simulink model "T5_button_controllable"  (R2022b)
settings: Solver=FixedStepAuto  StartTime=0.0  StopTime=96  FixedStep=0.01  RelTol=1e-3
undefined symbols (not defined in the file): cableArea, High, Low, Scaling_factor, Ts, Vnom
libraries: fl_lib x145, nesl_utility x56, simulink x54, ee_lib x4
(part 1 of 3)
settings Model: Creator=mingreico  LastModifiedBy=mingreico

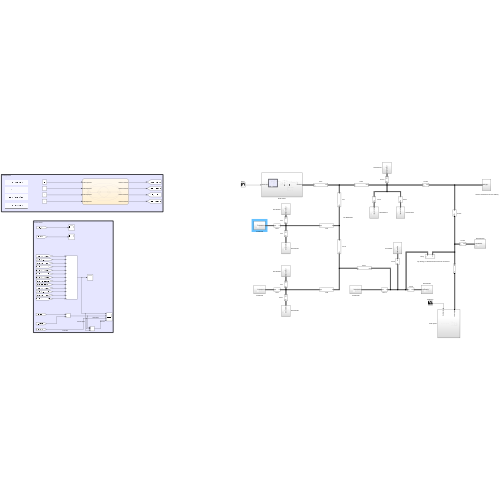
[thumbnail: Simulink's stored preview of the top-level diagram]
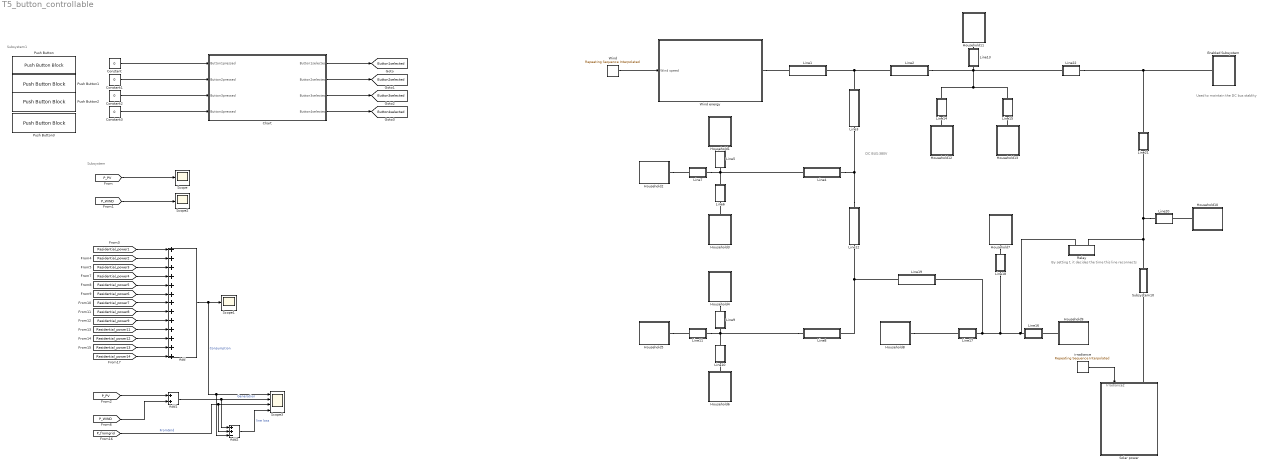
== system T5_button_controllable ==
  note: Subsystem
  note: Subsystem1
  note: By setting t, it decides the time this line reconnects
  note: Used to maintain the DC bus stablity
  note: DC BUS:380V
  Add : Sum  Inputs=+++++++++++++
  Add1 : Sum
  Add2 : Sum  Inputs=++-
  Chart : Stateflow chart  TreatAsAtomicUnit=on
  Constant{,1..3} (4 alike) : Constant  Value=0  OutDataTypeStr=boolean
  Enabled Subsystem : Subsystem
  Household1 : Subsystem
  Household10 : Subsystem
  Household11 : Subsystem
  Household12 : Subsystem
  Household13 : Subsystem
  Household2 : Subsystem
  Household3 : Subsystem
  Household4 : Subsystem
  Household5 : Subsystem
  Household6 : Subsystem
  Household7 : Subsystem
  Household8 : Subsystem
  Household9 : Subsystem
  Line1 : Subsystem  mask{rho=1.68e-8, l=2.0, A=cableArea}
      mask prompts: rho "Specific resistivity in Ohm*m"; l "Length in m"; A "Cross sectional area in m^2"
  Line10 : Subsystem  mask{rho=1.68e-8, l=2.0, A=cableArea}
      mask prompts: rho "Specific resistivity in Ohm*m"; l "Length in m"; A "Cross sectional area in m^2"
  Line11 : Subsystem  mask{rho=1.68e-8, l=2.0, A=cableArea}
      mask prompts: rho "Specific resistivity in Ohm*m"; l "Length in m"; A "Cross sectional area in m^2"
  Line12 : Subsystem  mask{rho=1.68e-8, l=2.0, A=cableArea}
      mask prompts: rho "Specific resistivity in Ohm*m"; l "Length in m"; A "Cross sectional area in m^2"
  Line13 : Subsystem  mask{rho=1.68e-8, l=2.0, A=cableArea}
      mask prompts: rho "Specific resistivity in Ohm*m"; l "Length in m"; A "Cross sectional area in m^2"
  Line14 : Subsystem  mask{rho=1.68e-8, l=2.0, A=cableArea}
      mask prompts: rho "Specific resistivity in Ohm*m"; l "Length in m"; A "Cross sectional area in m^2"
  Line15 : Subsystem  mask{rho=1.68e-8, l=2.0, A=cableArea}
      mask prompts: rho "Specific resistivity in Ohm*m"; l "Length in m"; A "Cross sectional area in m^2"
  Line16 : Subsystem  mask{rho=1.68e-8, l=2.0, A=cableArea}
      mask prompts: rho "Specific resistivity in Ohm*m"; l "Length in m"; A "Cross sectional area in m^2"
  Line17 : Subsystem  mask{rho=1.68e-8, l=2.0, A=cableArea}
      mask prompts: rho "Specific resistivity in Ohm*m"; l "Length in m"; A "Cross sectional area in m^2"
  Line18 : Subsystem  mask{rho=1.68e-8, l=2.0, A=cableArea}
      mask prompts: rho "Specific resistivity in Ohm*m"; l "Length in m"; A "Cross sectional area in m^2"
  Line19 : Subsystem  mask{rho=1.68e-8, l=2.0, A=cableArea}
      mask prompts: rho "Specific resistivity in Ohm*m"; l "Length in m"; A "Cross sectional area in m^2"
  Line2 : Subsystem  mask{rho=1.68e-8, l=2.0, A=cableArea}
      mask prompts: rho "Specific resistivity in Ohm*m"; l "Length in m"; A "Cross sectional area in m^2"
  Line20 : Subsystem  mask{rho=1.68e-8, l=2.0, A=cableArea}
      mask prompts: rho "Specific resistivity in Ohm*m"; l "Length in m"; A "Cross sectional area in m^2"
  Line21 : Subsystem  mask{rho=1.68e-8, l=2.0, A=cableArea}
      mask prompts: rho "Specific resistivity in Ohm*m"; l "Length in m"; A "Cross sectional area in m^2"
  Line22 : Subsystem  mask{rho=1.68e-8, l=2.0, A=cableArea}
      mask prompts: rho "Specific resistivity in Ohm*m"; l "Length in m"; A "Cross sectional area in m^2"
  Line3 : Subsystem  mask{rho=1.68e-8, l=2.0, A=cableArea}
      mask prompts: rho "Specific resistivity in Ohm*m"; l "Length in m"; A "Cross sectional area in m^2"
  Line4 : Subsystem  mask{rho=1.68e-8, l=2.0, A=cableArea}
      mask prompts: rho "Specific resistivity in Ohm*m"; l "Length in m"; A "Cross sectional area in m^2"
  Line5 : Subsystem  mask{rho=1.68e-8, l=2.0, A=cableArea}
      mask prompts: rho "Specific resistivity in Ohm*m"; l "Length in m"; A "Cross sectional area in m^2"
  Line6 : Subsystem  mask{rho=1.68e-8, l=2.0, A=cableArea}
      mask prompts: rho "Specific resistivity in Ohm*m"; l "Length in m"; A "Cross sectional area in m^2"
  Line7 : Subsystem  mask{rho=1.68e-8, l=2.0, A=cableArea}
      mask prompts: rho "Specific resistivity in Ohm*m"; l "Length in m"; A "Cross sectional area in m^2"
  Line8 : Subsystem  mask{rho=1.68e-8, l=2.0, A=cableArea}
      mask prompts: rho "Specific resistivity in Ohm*m"; l "Length in m"; A "Cross sectional area in m^2"
  Line9 : Subsystem  mask{rho=1.68e-8, l=2.0, A=cableArea}
      mask prompts: rho "Specific resistivity in Ohm*m"; l "Length in m"; A "Cross sectional area in m^2"
  Push Button : PushButtonBlock  ButtonText=Button_SpringAllday  OffValue=0.000000
  Push Button1 : PushButtonBlock  ButtonText=Button_SummerAllday  OffValue=0.000000
  Push Button2 : PushButtonBlock  ButtonText=Button_AutumnAllday  OffValue=0.000000
  Push Button3 : PushButtonBlock  ButtonText=Button_WinterAllday  OffValue=0.000000
  Relay : Subsystem  mask{t=140}
      mask prompts: t "Specific jumping time"
  Scope : Scope
  Scope1 : Scope
  Scope2 : Scope
  Scope3 : Scope  NumInputPorts=4
  Solar power : Subsystem
  Subsystem10 : Subsystem  mask{rho=1.68e-8, l=2.0, A=cableArea}
      mask prompts: rho "Specific resistivity in Ohm*m"; l "Length in m"; A "Cross sectional area in m^2"
  "Wind  " : simulink/Sources/Repeating Sequence Interpolated  OutValues=[6 5 5 8 10 11 17 20 22 29 31 36 34 37 37 37 32 30 29 22 15 11 9 13]*0.7  TimeValues=[0 1 2 3 4 5 6 7 8 9 10 11 12 13 14 15 16 17 18 19 20 21 22 23]  LookUpMeth=Interpolation-Use End Values  tsamp=0.01  OutMin=[]  OutMax=[]  OutDataTypeStr=double  OutputDataTypeScalingMode=double  OutDataType=fixdt(0,8)  OutScaling=2^-10
  Wind energy : Subsystem
  "irradiance " : simulink/Sources/Repeating Sequence Interpolated  OutValues=[0 0 0 0 0 0 43 163 310 464 601 707 776 810 807 769 696 594 469 331 189 52 0 0]  TimeValues=[0 1 2 3 4 5 6 7 8 9 10 11 12 13 14 15 16 17 18 19 20 21 22 23]  LookUpMeth=Interpolation-Use End Values  tsamp=0.01  OutMin=[]  OutMax=[]  OutDataTypeStr=double  OutputDataTypeScalingMode=double  OutDataType=fixdt(0,8)  OutScaling=2^-10
  tag scope: Button1selected=global, Button2selected=global, Button3selected=global, Button4selected=global
  wires:
  Constant3/1 -> Chart/4(Button4pressed)
  Constant2/1 -> Chart/3(Button3pressed)
  Constant1/1 -> Chart/2(Button2pressed)
  Constant/1 -> Chart/1(Button1pressed)
  Chart/4(" Button4selected") -> [Button4selected]
  Chart/3(" Button3selected") -> [Button3selected]
  Chart/2(" Button2selected") -> [Button2selected]
  Chart/1(" Button1selected") -> [Button1selected]
  Add1/1 -> Add2/1, Scope3/2  "Generation"
  [P_WIND] -> Add1/2
  [P_PV] -> Add1/1
  Add/1 -> Scope1/1, Add2/3, Scope3/1  "Consumption"
  [Residential_power13] -> Add/12
  [Residential_power12] -> Add/11
  [Residential_power11] -> Add/10
  [Residential_power9] -> Add/9
  [Residential_power8] -> Add/8
  [Residential_power7] -> Add/7
  [Residential_power6] -> Add/6
  [Residential_power5] -> Add/5
  [Residential_power4] -> Add/4
  [Residential_power3] -> Add/3
  [Residential_power2] -> Add/2
  [Residential_power1] -> Add/1
  [P_WIND] -> Scope2/1
  [P_PV] -> Scope/1
  [P_fromgrid] -> Add2/2, Scope3/3  "FromGrid"
  [Residential_power14] -> Add/13
  Add2/1 -> Scope3/4  "line loss"
  "irradiance "/1 -> Solar power/1(Irradiance2)
  "Wind  "/1 -> Wind energy/1(Wind speed)
  connections:
  Line8/RConn1 -- Line9/LConn1 -- Line10/RConn1 -- Line11/LConn1
  Line2/RConn1 -- Line14/LConn1 -- Line15/LConn1 -- Line22/LConn1 -- Line13/LConn1
  Line20/LConn1 -- Relay/LConn2 -- Subsystem10/RConn1 -- Line21/RConn1
  Line1/RConn1 -- Line2/LConn1 -- Line3/LConn1
  Line8/LConn1 -- Line12/RConn1 -- Line19/LConn1
  Line16/LConn1 -- Line18/LConn1 -- Line17/LConn1 -- Line19/RConn1 -- Relay/LConn1
  Line21/LConn1 -- Enabled Subsystem/RConn1 -- Line22/RConn1
  Line12/LConn1 -- Line3/RConn1 -- Line4/LConn1
  Line7/LConn1 -- Line5/LConn1 -- Line4/RConn1 -- Line6/RConn1
  Household12/RConn1 -- Line14/RConn1
  Household1/RConn1 -- Line5/RConn1
  Household13/RConn1 -- Line15/RConn1
  Household7/RConn1 -- Line18/RConn1
  Household6/RConn1 -- Line10/LConn1
  Household9/RConn1 -- Line16/RConn1
  Household8/RConn1 -- Line17/RConn1
  Household11/RConn1 -- Line13/RConn1
  Household5/RConn1 -- Line11/RConn1
  Household2/RConn1 -- Line7/RConn1
  Household4/RConn1 -- Line9/RConn1
  Household3/RConn1 -- Line6/LConn1
  Household10/RConn1 -- Line20/RConn1
  Wind energy/RConn1 -- Line1/LConn1
  Solar power/LConn1 -- Subsystem10/LConn1

== system T5_button_controllable/Enabled Subsystem ==
  Average-Value DC-DC Converter : ee_lib/Semiconductors & Converters/Converters/Average-Value DC-DC Converter  control_option=ee.enum.converters.controlinput.voltage  converter_type=ee.enum.converters.dcdctype.buck  efficiency_option=ee.enum.converters.efficiency.constant  efficiency_fixed=100  i_vec=[0, 2, 5] A  efficiency_vec=[90, 95, 98]
      settings: InternalSimscapePortConfiguration="{\"Bottom\":[],\"Left\":[{\"id\":\"Vref\",\"label\":\"Vref\",\"type\":\"input\"},{\"id\":\"p1\",\"label\":\"1+\",\"type\":\"foundation.electrical.electrical\"},{\"id\":\"n1\",\"label\":\"1-\",\"type\":\"foundation.electrical.electrical\"}],\"Right\":[{\"id\":\"p2\",\"label\":\"2+\",\"type\":\"foundation.electrical.electrical\"},{\"id\":\"n2\",\"label\":\"2-\",\"type\":\"foundation.electrical.electrical\"}],\"Top\":[]}"
  Constant : Constant  Value=Vnom
  Current Sensor : fl_lib/Electrical/Electrical Sensors/Current Sensor
  PS-Simulink Converter : nesl_utility/PS-Simulink Converter  PhysicalDomain=network_engine_domain  SubClassName=ps_output  LeftPortType=input  RightPortType=output  PseudoPeriodic=off  Frequencies=[]  VectorFormat=inherit  Unit=inherit  AffineConversion=off
  PS-Simulink Converter1 : nesl_utility/PS-Simulink Converter  PhysicalDomain=network_engine_domain  SubClassName=ps_output  LeftPortType=input  RightPortType=output  PseudoPeriodic=off  Frequencies=[]  VectorFormat=inherit  Unit=inherit  AffineConversion=off
  Product : Product
  Scope : Scope
  Simscape Bus1 : SimscapeBus  HierarchyStrings=High;Low
  Simulink-PS Converter : nesl_utility/Simulink-PS Converter  PhysicalDomain=network_engine_domain  SubClassName=ps_input  LeftPortType=input  RightPortType=output  PseudoPeriodic=off  Frequencies=[]  NoiseDistribution=none  NoiseParameters=[]  Unit=1  AffineConversion=off  FilteringAndDerivatives=provide  SimscapeFilterOrder=1  InputFilterTimeConstant=0.001  UdotUserProvided=0
  Voltage Sensor : fl_lib/Electrical/Electrical Sensors/Voltage Sensor
  Voltage Source : ee_lib/Sources/Voltage Source  dc_voltage=1000 V  ac_voltage=0 V  ac_shift=0 rad  ac_frequency=60 Hz  noise_mode=ee.enum.sources.noise.Disabled  PSD=0 V^2/Hz  sample_time=1e-3 s  repeatability=ee.enum.sources.repeatability.NotRepeatable  user_seed=0  auto_seed=3499211588  i_specify=off  i_priority=None  i=0 A  i_nominal_specify=off  i_nominal_unit=A  i_nominal_value=1  v_specify=off  v_priority=None  v=0 V  v_nominal_specify=off  v_nominal_unit=V  v_nominal_value=1
  Maingrid : PMIOPort  Side=Right
  tag scope: P_fromgrid=global
  wires:
  Constant/1 -> Simulink-PS Converter/1
  PS-Simulink Converter/1 -> Scope/1, Product/1
  PS-Simulink Converter1/1 -> Product/2
  Product/1 -> [P_fromgrid]
  connections:
  Maingrid/RConn1 -- Simscape Bus1/RConn1
  Voltage Source/LConn1 -- Average-Value DC-DC Converter/LConn2
  Voltage Source/RConn1 -- Average-Value DC-DC Converter/LConn3
  Simulink-PS Converter/RConn1 -- Average-Value DC-DC Converter/LConn1
  Average-Value DC-DC Converter/RConn2 -- Voltage Sensor/RConn2 -- Simscape Bus1/LConn2
  Current Sensor/RConn2 -- Voltage Sensor/LConn1 -- Simscape Bus1/LConn1
  Current Sensor/LConn1 -- Average-Value DC-DC Converter/RConn1
  PS-Simulink Converter1/LConn1 -- Voltage Sensor/RConn1
  PS-Simulink Converter/LConn1 -- Current Sensor/RConn1

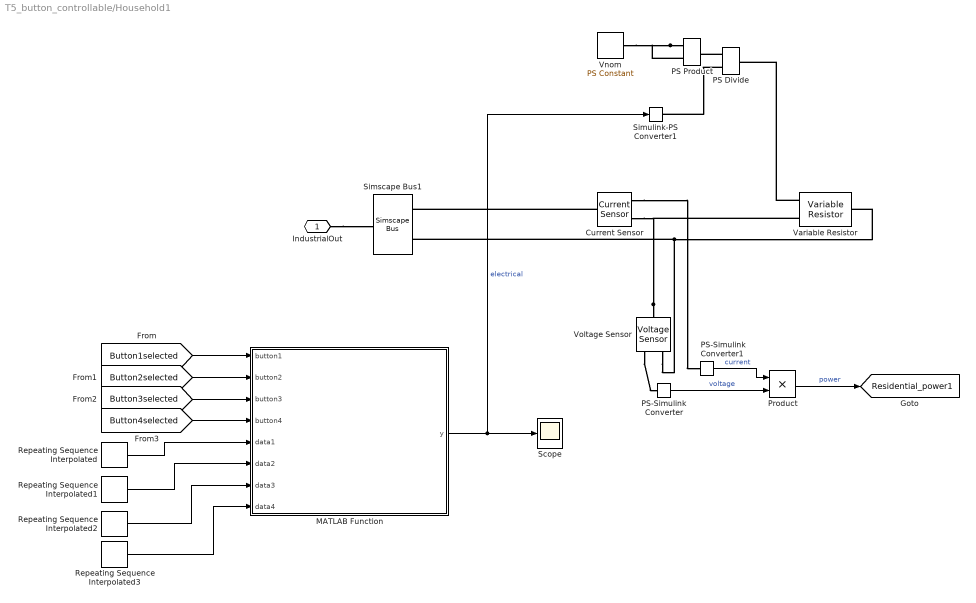
== system T5_button_controllable/Household1 ==
  Current Sensor : fl_lib/Electrical/Electrical Sensors/Current Sensor
  MATLAB Function : MATLAB Function  TreatAsAtomicUnit=on
  PS Divide : fl_lib/Physical Signals/Functions/PS Divide
  PS Product : fl_lib/Physical Signals/Functions/PS Product
  PS-Simulink Converter : nesl_utility/PS-Simulink Converter  PhysicalDomain=network_engine_domain  SubClassName=ps_output  LeftPortType=input  RightPortType=output  PseudoPeriodic=off  Frequencies=[]  VectorFormat=inherit  Unit=inherit  AffineConversion=off
  PS-Simulink Converter1 : nesl_utility/PS-Simulink Converter  PhysicalDomain=network_engine_domain  SubClassName=ps_output  LeftPortType=input  RightPortType=output  PseudoPeriodic=off  Frequencies=[]  VectorFormat=inherit  Unit=inherit  AffineConversion=off
  Product : Product
  Repeating Sequence Interpolated : simulink/Sources/Repeating Sequence Interpolated  OutValues=Household3_Springallday  TimeValues=Allday_timevector  LookUpMeth=Interpolation-Use End Values  tsamp=0.01  OutMin=[]  OutMax=[]  OutDataTypeStr=double  OutputDataTypeScalingMode=double  OutDataType=fixdt(0,8)  OutScaling=2^-10
  Repeating Sequence Interpolated1 : simulink/Sources/Repeating Sequence Interpolated  OutValues=Household3_Summerallday  TimeValues=Allday_timevector  LookUpMeth=Interpolation-Use End Values  tsamp=0.01  OutMin=[]  OutMax=[]  OutDataTypeStr=double  OutputDataTypeScalingMode=double  OutDataType=fixdt(0,8)  OutScaling=2^-10
  Repeating Sequence Interpolated2 : simulink/Sources/Repeating Sequence Interpolated  OutValues=Household3_Autumnallday  TimeValues=Allday_timevector  LookUpMeth=Interpolation-Use End Values  tsamp=0.01  OutMin=[]  OutMax=[]  OutDataTypeStr=double  OutputDataTypeScalingMode=double  OutDataType=fixdt(0,8)  OutScaling=2^-10
  Repeating Sequence Interpolated3 : simulink/Sources/Repeating Sequence Interpolated  OutValues=Household3_Winterallday  TimeValues=Allday_timevector  LookUpMeth=Interpolation-Use End Values  tsamp=0.01  OutMin=[]  OutMax=[]  OutDataTypeStr=double  OutputDataTypeScalingMode=double  OutDataType=fixdt(0,8)  OutScaling=2^-10
  Scope : Scope
  Simscape Bus1 : SimscapeBus  HierarchyStrings=High;Low
  Simulink-PS Converter1 : nesl_utility/Simulink-PS Converter  PhysicalDomain=network_engine_domain  SubClassName=ps_input  LeftPortType=input  RightPortType=output  PseudoPeriodic=off  Frequencies=[]  NoiseDistribution=none  NoiseParameters=[]  Unit=V*A  AffineConversion=off  FilteringAndDerivatives=provide  SimscapeFilterOrder=1  InputFilterTimeConstant=0.001  UdotUserProvided=0
  Variable Resistor : fl_lib/Electrical/Electrical Elements/Variable Resistor  Rmin=0 Ohm  i_specify=off  i_priority=None  i=0 A  i_nominal_specify=off  i_nominal_unit=A  i_nominal_value=1  v_specify=off  v_priority=None  v=0 V  v_nominal_specify=off  v_nominal_unit=V  v_nominal_value=1
  Vnom : fl_lib/Physical Signals/Sources/PS Constant  constant=Vnom V
  Voltage Sensor : fl_lib/Electrical/Electrical Sensors/Voltage Sensor
  IndustrialOut : PMIOPort  Side=Right
  tag scope: Residential_power1=global
  wires:
  MATLAB Function/1(y) -> Simulink-PS Converter1/1, Scope/1  "electrical"
  PS-Simulink Converter/1 -> Product/2  "voltage"
  PS-Simulink Converter1/1 -> Product/1  "current"
  Product/1 -> [Residential_power1]  "power"
  [Button4selected] -> MATLAB Function/4(button4)
  [Button3selected] -> MATLAB Function/3(button3)
  [Button2selected] -> MATLAB Function/2(button2)
  [Button1selected] -> MATLAB Function/1(button1)
  Repeating Sequence Interpolated/1 -> MATLAB Function/5(data1)
  Repeating Sequence Interpolated1/1 -> MATLAB Function/6(data2)
  Repeating Sequence Interpolated2/1 -> MATLAB Function/7(data3)
  Repeating Sequence Interpolated3/1 -> MATLAB Function/8(data4)
  connections:
  PS Divide/LConn1 -- PS Product/RConn1
  Variable Resistor/LConn1 -- PS Divide/RConn1
  PS Divide/LConn2 -- Simulink-PS Converter1/RConn1
  PS Product/LConn1 -- PS Product/LConn2 -- Vnom/RConn1
  Voltage Sensor/RConn2 -- Variable Resistor/RConn1 -- Simscape Bus1/LConn2
  IndustrialOut/RConn1 -- Simscape Bus1/RConn1
  Voltage Sensor/LConn1 -- Variable Resistor/LConn2 -- Current Sensor/RConn2
  Voltage Sensor/RConn1 -- PS-Simulink Converter/LConn1
  Current Sensor/RConn1 -- PS-Simulink Converter1/LConn1
  Current Sensor/LConn1 -- Simscape Bus1/LConn1

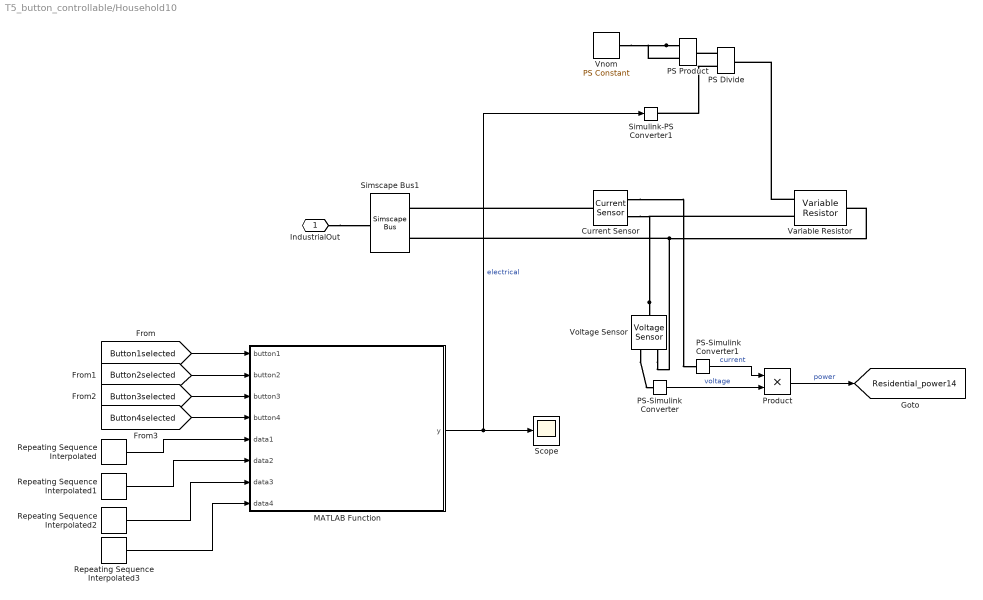
== system T5_button_controllable/Household10 ==
  Current Sensor : fl_lib/Electrical/Electrical Sensors/Current Sensor
  MATLAB Function : MATLAB Function  TreatAsAtomicUnit=on
  PS Divide : fl_lib/Physical Signals/Functions/PS Divide
  PS Product : fl_lib/Physical Signals/Functions/PS Product
  PS-Simulink Converter : nesl_utility/PS-Simulink Converter  PhysicalDomain=network_engine_domain  SubClassName=ps_output  LeftPortType=input  RightPortType=output  PseudoPeriodic=off  Frequencies=[]  VectorFormat=inherit  Unit=inherit  AffineConversion=off
  PS-Simulink Converter1 : nesl_utility/PS-Simulink Converter  PhysicalDomain=network_engine_domain  SubClassName=ps_output  LeftPortType=input  RightPortType=output  PseudoPeriodic=off  Frequencies=[]  VectorFormat=inherit  Unit=inherit  AffineConversion=off
  Product : Product
  Repeating Sequence Interpolated : simulink/Sources/Repeating Sequence Interpolated  OutValues=Household14_Springallday  TimeValues=Allday_timevector  LookUpMeth=Interpolation-Use End Values  tsamp=0.01  OutMin=[]  OutMax=[]  OutDataTypeStr=double  OutputDataTypeScalingMode=double  OutDataType=fixdt(0,8)  OutScaling=2^-10
  Repeating Sequence Interpolated1 : simulink/Sources/Repeating Sequence Interpolated  OutValues=Household14_Summerallday  TimeValues=Allday_timevector  LookUpMeth=Interpolation-Use End Values  tsamp=0.01  OutMin=[]  OutMax=[]  OutDataTypeStr=double  OutputDataTypeScalingMode=double  OutDataType=fixdt(0,8)  OutScaling=2^-10
  Repeating Sequence Interpolated2 : simulink/Sources/Repeating Sequence Interpolated  OutValues=Household14_Autumnallday  TimeValues=Allday_timevector  LookUpMeth=Interpolation-Use End Values  tsamp=0.01  OutMin=[]  OutMax=[]  OutDataTypeStr=double  OutputDataTypeScalingMode=double  OutDataType=fixdt(0,8)  OutScaling=2^-10
  Repeating Sequence Interpolated3 : simulink/Sources/Repeating Sequence Interpolated  OutValues=Household14_Winterallday  TimeValues=Allday_timevector  LookUpMeth=Interpolation-Use End Values  tsamp=0.01  OutMin=[]  OutMax=[]  OutDataTypeStr=double  OutputDataTypeScalingMode=double  OutDataType=fixdt(0,8)  OutScaling=2^-10
  Scope : Scope
  Simscape Bus1 : SimscapeBus  HierarchyStrings=High;Low
  Simulink-PS Converter1 : nesl_utility/Simulink-PS Converter  PhysicalDomain=network_engine_domain  SubClassName=ps_input  LeftPortType=input  RightPortType=output  PseudoPeriodic=off  Frequencies=[]  NoiseDistribution=none  NoiseParameters=[]  Unit=V*A  AffineConversion=off  FilteringAndDerivatives=provide  SimscapeFilterOrder=1  InputFilterTimeConstant=0.001  UdotUserProvided=0
  Variable Resistor : fl_lib/Electrical/Electrical Elements/Variable Resistor  Rmin=0 Ohm  i_specify=off  i_priority=None  i=0 A  i_nominal_specify=off  i_nominal_unit=A  i_nominal_value=1  v_specify=off  v_priority=None  v=0 V  v_nominal_specify=off  v_nominal_unit=V  v_nominal_value=1
  Vnom : fl_lib/Physical Signals/Sources/PS Constant  constant=Vnom V
  Voltage Sensor : fl_lib/Electrical/Electrical Sensors/Voltage Sensor
  IndustrialOut : PMIOPort  Side=Right
  tag scope: Residential_power14=global
  wires:
  MATLAB Function/1(y) -> Scope/1, Simulink-PS Converter1/1  "electrical"
  PS-Simulink Converter/1 -> Product/2  "voltage"
  PS-Simulink Converter1/1 -> Product/1  "current"
  Product/1 -> [Residential_power14]  "power"
  [Button4selected] -> MATLAB Function/4(button4)
  [Button3selected] -> MATLAB Function/3(button3)
  [Button2selected] -> MATLAB Function/2(button2)
  [Button1selected] -> MATLAB Function/1(button1)
  Repeating Sequence Interpolated/1 -> MATLAB Function/5(data1)
  Repeating Sequence Interpolated1/1 -> MATLAB Function/6(data2)
  Repeating Sequence Interpolated2/1 -> MATLAB Function/7(data3)
  Repeating Sequence Interpolated3/1 -> MATLAB Function/8(data4)
  connections:
  PS Divide/LConn1 -- PS Product/RConn1
  Variable Resistor/LConn1 -- PS Divide/RConn1
  PS Divide/LConn2 -- Simulink-PS Converter1/RConn1
  PS Product/LConn1 -- PS Product/LConn2 -- Vnom/RConn1
  Voltage Sensor/RConn2 -- Simscape Bus1/LConn2 -- Variable Resistor/RConn1
  IndustrialOut/RConn1 -- Simscape Bus1/RConn1
  Voltage Sensor/LConn1 -- Variable Resistor/LConn2 -- Current Sensor/RConn2
  Voltage Sensor/RConn1 -- PS-Simulink Converter/LConn1
  Current Sensor/RConn1 -- PS-Simulink Converter1/LConn1
  Current Sensor/LConn1 -- Simscape Bus1/LConn1

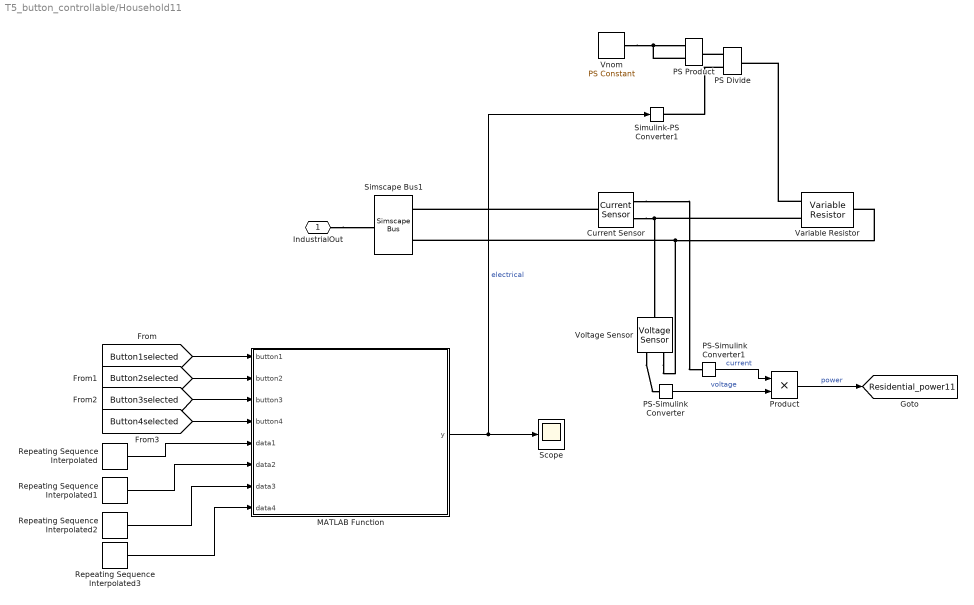
== system T5_button_controllable/Household11 ==
  Current Sensor : fl_lib/Electrical/Electrical Sensors/Current Sensor
  MATLAB Function : MATLAB Function  TreatAsAtomicUnit=on
  PS Divide : fl_lib/Physical Signals/Functions/PS Divide
  PS Product : fl_lib/Physical Signals/Functions/PS Product
  PS-Simulink Converter : nesl_utility/PS-Simulink Converter  PhysicalDomain=network_engine_domain  SubClassName=ps_output  LeftPortType=input  RightPortType=output  PseudoPeriodic=off  Frequencies=[]  VectorFormat=inherit  Unit=inherit  AffineConversion=off
  PS-Simulink Converter1 : nesl_utility/PS-Simulink Converter  PhysicalDomain=network_engine_domain  SubClassName=ps_output  LeftPortType=input  RightPortType=output  PseudoPeriodic=off  Frequencies=[]  VectorFormat=inherit  Unit=inherit  AffineConversion=off
  Product : Product
  Repeating Sequence Interpolated : simulink/Sources/Repeating Sequence Interpolated  OutValues=Household7_Springallday  TimeValues=Allday_timevector  LookUpMeth=Interpolation-Use End Values  tsamp=0.01  OutMin=[]  OutMax=[]  OutDataTypeStr=double  OutputDataTypeScalingMode=double  OutDataType=fixdt(0,8)  OutScaling=2^-10
  Repeating Sequence Interpolated1 : simulink/Sources/Repeating Sequence Interpolated  OutValues=Household7_Summerallday  TimeValues=Allday_timevector  LookUpMeth=Interpolation-Use End Values  tsamp=0.01  OutMin=[]  OutMax=[]  OutDataTypeStr=double  OutputDataTypeScalingMode=double  OutDataType=fixdt(0,8)  OutScaling=2^-10
  Repeating Sequence Interpolated2 : simulink/Sources/Repeating Sequence Interpolated  OutValues=Household7_Autumnallday  TimeValues=Allday_timevector  LookUpMeth=Interpolation-Use End Values  tsamp=0.01  OutMin=[]  OutMax=[]  OutDataTypeStr=double  OutputDataTypeScalingMode=double  OutDataType=fixdt(0,8)  OutScaling=2^-10
  Repeating Sequence Interpolated3 : simulink/Sources/Repeating Sequence Interpolated  OutValues=Household7_Winterallday  TimeValues=Allday_timevector  LookUpMeth=Interpolation-Use End Values  tsamp=0.01  OutMin=[]  OutMax=[]  OutDataTypeStr=double  OutputDataTypeScalingMode=double  OutDataType=fixdt(0,8)  OutScaling=2^-10
  Scope : Scope
  Simscape Bus1 : SimscapeBus  HierarchyStrings=High;Low
  Simulink-PS Converter1 : nesl_utility/Simulink-PS Converter  PhysicalDomain=network_engine_domain  SubClassName=ps_input  LeftPortType=input  RightPortType=output  PseudoPeriodic=off  Frequencies=[]  NoiseDistribution=none  NoiseParameters=[]  Unit=V*A  AffineConversion=off  FilteringAndDerivatives=provide  SimscapeFilterOrder=1  InputFilterTimeConstant=0.001  UdotUserProvided=0
  Variable Resistor : fl_lib/Electrical/Electrical Elements/Variable Resistor  Rmin=0 Ohm  i_specify=off  i_priority=None  i=0 A  i_nominal_specify=off  i_nominal_unit=A  i_nominal_value=1  v_specify=off  v_priority=None  v=0 V  v_nominal_specify=off  v_nominal_unit=V  v_nominal_value=1
  Vnom : fl_lib/Physical Signals/Sources/PS Constant  constant=Vnom V
  Voltage Sensor : fl_lib/Electrical/Electrical Sensors/Voltage Sensor
  IndustrialOut : PMIOPort  Side=Right
  tag scope: Residential_power11=global
  wires:
  Repeating Sequence Interpolated3/1 -> MATLAB Function/8(data4)
  Repeating Sequence Interpolated2/1 -> MATLAB Function/7(data3)
  Repeating Sequence Interpolated1/1 -> MATLAB Function/6(data2)
  Repeating Sequence Interpolated/1 -> MATLAB Function/5(data1)
  [Button1selected] -> MATLAB Function/1(button1)
  [Button2selected] -> MATLAB Function/2(button2)
  [Button3selected] -> MATLAB Function/3(button3)
  [Button4selected] -> MATLAB Function/4(button4)
  Product/1 -> [Residential_power11]  "power"
  PS-Simulink Converter1/1 -> Product/1  "current"
  PS-Simulink Converter/1 -> Product/2  "voltage"
  MATLAB Function/1(y) -> Simulink-PS Converter1/1, Scope/1  "electrical"
  connections:
  Current Sensor/LConn1 -- Simscape Bus1/LConn1
  Current Sensor/RConn1 -- PS-Simulink Converter1/LConn1
  Voltage Sensor/RConn1 -- PS-Simulink Converter/LConn1
  Current Sensor/RConn2 -- Variable Resistor/LConn2 -- Voltage Sensor/LConn1
  IndustrialOut/RConn1 -- Simscape Bus1/RConn1
  Variable Resistor/RConn1 -- Simscape Bus1/LConn2 -- Voltage Sensor/RConn2
  Vnom/RConn1 -- PS Product/LConn2 -- PS Product/LConn1
  PS Divide/LConn2 -- Simulink-PS Converter1/RConn1
  Variable Resistor/LConn1 -- PS Divide/RConn1
  PS Divide/LConn1 -- PS Product/RConn1

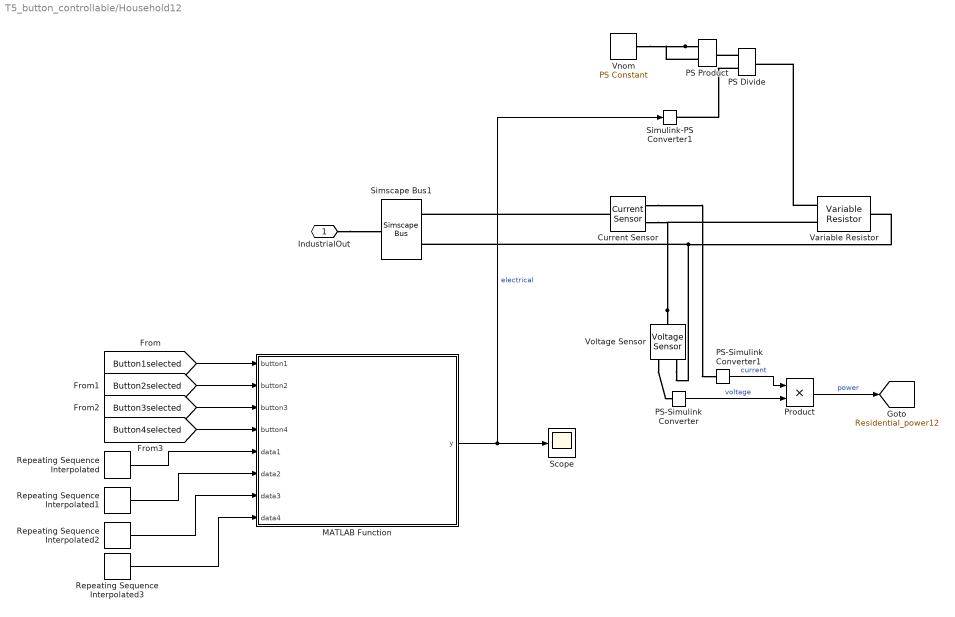
== system T5_button_controllable/Household12 ==
  Current Sensor : fl_lib/Electrical/Electrical Sensors/Current Sensor
  MATLAB Function : MATLAB Function  TreatAsAtomicUnit=on
  PS Divide : fl_lib/Physical Signals/Functions/PS Divide
  PS Product : fl_lib/Physical Signals/Functions/PS Product
  PS-Simulink Converter : nesl_utility/PS-Simulink Converter  PhysicalDomain=network_engine_domain  SubClassName=ps_output  LeftPortType=input  RightPortType=output  PseudoPeriodic=off  Frequencies=[]  VectorFormat=inherit  Unit=inherit  AffineConversion=off
  PS-Simulink Converter1 : nesl_utility/PS-Simulink Converter  PhysicalDomain=network_engine_domain  SubClassName=ps_output  LeftPortType=input  RightPortType=output  PseudoPeriodic=off  Frequencies=[]  VectorFormat=inherit  Unit=inherit  AffineConversion=off
  Product : Product
  Repeating Sequence Interpolated : simulink/Sources/Repeating Sequence Interpolated  OutValues=Household11_Springallday  TimeValues=Allday_timevector  LookUpMeth=Interpolation-Use End Values  tsamp=0.01  OutMin=[]  OutMax=[]  OutDataTypeStr=double  OutputDataTypeScalingMode=double  OutDataType=fixdt(0,8)  OutScaling=2^-10
  Repeating Sequence Interpolated1 : simulink/Sources/Repeating Sequence Interpolated  OutValues=Household11_Summerallday  TimeValues=Allday_timevector  LookUpMeth=Interpolation-Use End Values  tsamp=0.01  OutMin=[]  OutMax=[]  OutDataTypeStr=double  OutputDataTypeScalingMode=double  OutDataType=fixdt(0,8)  OutScaling=2^-10
  Repeating Sequence Interpolated2 : simulink/Sources/Repeating Sequence Interpolated  OutValues=Household11_Autumnallday  TimeValues=Allday_timevector  LookUpMeth=Interpolation-Use End Values  tsamp=0.01  OutMin=[]  OutMax=[]  OutDataTypeStr=double  OutputDataTypeScalingMode=double  OutDataType=fixdt(0,8)  OutScaling=2^-10
  Repeating Sequence Interpolated3 : simulink/Sources/Repeating Sequence Interpolated  OutValues=Household11_Winterallday  TimeValues=Allday_timevector  LookUpMeth=Interpolation-Use End Values  tsamp=0.01  OutMin=[]  OutMax=[]  OutDataTypeStr=double  OutputDataTypeScalingMode=double  OutDataType=fixdt(0,8)  OutScaling=2^-10
  Scope : Scope
  Simscape Bus1 : SimscapeBus  HierarchyStrings=High;Low
  Simulink-PS Converter1 : nesl_utility/Simulink-PS Converter  PhysicalDomain=network_engine_domain  SubClassName=ps_input  LeftPortType=input  RightPortType=output  PseudoPeriodic=off  Frequencies=[]  NoiseDistribution=none  NoiseParameters=[]  Unit=V*A  AffineConversion=off  FilteringAndDerivatives=provide  SimscapeFilterOrder=1  InputFilterTimeConstant=0.001  UdotUserProvided=0
  Variable Resistor : fl_lib/Electrical/Electrical Elements/Variable Resistor  Rmin=0 Ohm  i_specify=off  i_priority=None  i=0 A  i_nominal_specify=off  i_nominal_unit=A  i_nominal_value=1  v_specify=off  v_priority=None  v=0 V  v_nominal_specify=off  v_nominal_unit=V  v_nominal_value=1
  Vnom : fl_lib/Physical Signals/Sources/PS Constant  constant=Vnom V
  Voltage Sensor : fl_lib/Electrical/Electrical Sensors/Voltage Sensor
  IndustrialOut : PMIOPort  Side=Right
  tag scope: Residential_power12=global
  wires:
  MATLAB Function/1(y) -> Simulink-PS Converter1/1, Scope/1  "electrical"
  PS-Simulink Converter/1 -> Product/2  "voltage"
  PS-Simulink Converter1/1 -> Product/1  "current"
  Product/1 -> [Residential_power12]  "power"
  [Button4selected] -> MATLAB Function/4(button4)
  [Button3selected] -> MATLAB Function/3(button3)
  [Button2selected] -> MATLAB Function/2(button2)
  [Button1selected] -> MATLAB Function/1(button1)
  Repeating Sequence Interpolated/1 -> MATLAB Function/5(data1)
  Repeating Sequence Interpolated1/1 -> MATLAB Function/6(data2)
  Repeating Sequence Interpolated2/1 -> MATLAB Function/7(data3)
  Repeating Sequence Interpolated3/1 -> MATLAB Function/8(data4)
  connections:
  PS Divide/LConn1 -- PS Product/RConn1
  Variable Resistor/LConn1 -- PS Divide/RConn1
  PS Divide/LConn2 -- Simulink-PS Converter1/RConn1
  PS Product/LConn1 -- PS Product/LConn2 -- Vnom/RConn1
  Voltage Sensor/RConn2 -- Simscape Bus1/LConn2 -- Variable Resistor/RConn1
  IndustrialOut/RConn1 -- Simscape Bus1/RConn1
  Voltage Sensor/LConn1 -- Variable Resistor/LConn2 -- Current Sensor/RConn2
  Voltage Sensor/RConn1 -- PS-Simulink Converter/LConn1
  Current Sensor/RConn1 -- PS-Simulink Converter1/LConn1
  Current Sensor/LConn1 -- Simscape Bus1/LConn1

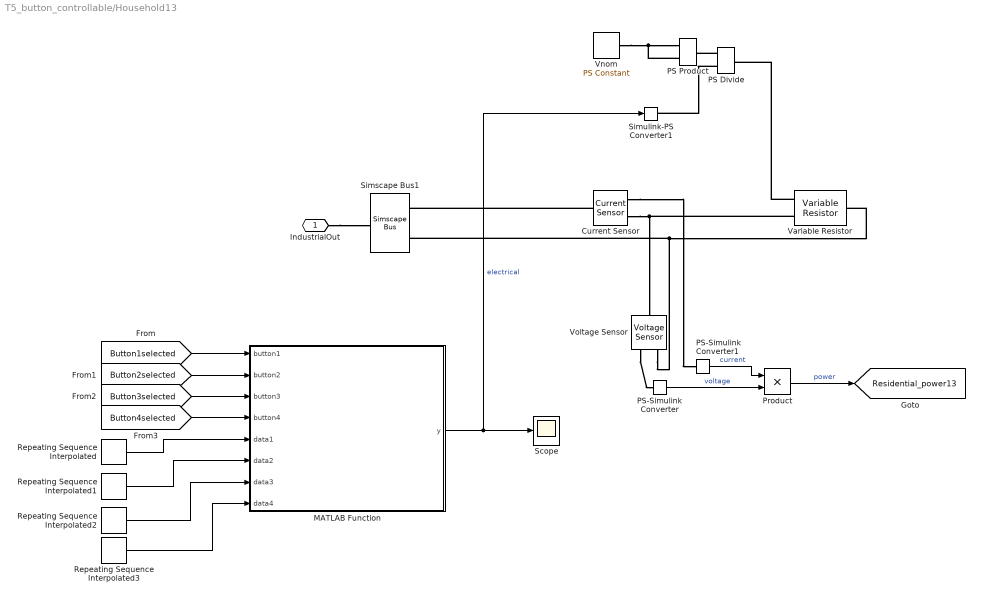
== system T5_button_controllable/Household13 ==
  Current Sensor : fl_lib/Electrical/Electrical Sensors/Current Sensor
  MATLAB Function : MATLAB Function  TreatAsAtomicUnit=on
  PS Divide : fl_lib/Physical Signals/Functions/PS Divide
  PS Product : fl_lib/Physical Signals/Functions/PS Product
  PS-Simulink Converter : nesl_utility/PS-Simulink Converter  PhysicalDomain=network_engine_domain  SubClassName=ps_output  LeftPortType=input  RightPortType=output  PseudoPeriodic=off  Frequencies=[]  VectorFormat=inherit  Unit=inherit  AffineConversion=off
  PS-Simulink Converter1 : nesl_utility/PS-Simulink Converter  PhysicalDomain=network_engine_domain  SubClassName=ps_output  LeftPortType=input  RightPortType=output  PseudoPeriodic=off  Frequencies=[]  VectorFormat=inherit  Unit=inherit  AffineConversion=off
  Product : Product
  Repeating Sequence Interpolated : simulink/Sources/Repeating Sequence Interpolated  OutValues=Household12_Springallday  TimeValues=Allday_timevector  LookUpMeth=Interpolation-Use End Values  tsamp=0.01  OutMin=[]  OutMax=[]  OutDataTypeStr=double  OutputDataTypeScalingMode=double  OutDataType=fixdt(0,8)  OutScaling=2^-10
  Repeating Sequence Interpolated1 : simulink/Sources/Repeating Sequence Interpolated  OutValues=Household12_Summerallday  TimeValues=Allday_timevector  LookUpMeth=Interpolation-Use End Values  tsamp=0.01  OutMin=[]  OutMax=[]  OutDataTypeStr=double  OutputDataTypeScalingMode=double  OutDataType=fixdt(0,8)  OutScaling=2^-10
  Repeating Sequence Interpolated2 : simulink/Sources/Repeating Sequence Interpolated  OutValues=Household12_Autumnallday  TimeValues=Allday_timevector  LookUpMeth=Interpolation-Use End Values  tsamp=0.01  OutMin=[]  OutMax=[]  OutDataTypeStr=double  OutputDataTypeScalingMode=double  OutDataType=fixdt(0,8)  OutScaling=2^-10
  Repeating Sequence Interpolated3 : simulink/Sources/Repeating Sequence Interpolated  OutValues=Household12_Winterallday  TimeValues=Allday_timevector  LookUpMeth=Interpolation-Use End Values  tsamp=0.01  OutMin=[]  OutMax=[]  OutDataTypeStr=double  OutputDataTypeScalingMode=double  OutDataType=fixdt(0,8)  OutScaling=2^-10
  Scope : Scope
  Simscape Bus1 : SimscapeBus  HierarchyStrings=High;Low
  Simulink-PS Converter1 : nesl_utility/Simulink-PS Converter  PhysicalDomain=network_engine_domain  SubClassName=ps_input  LeftPortType=input  RightPortType=output  PseudoPeriodic=off  Frequencies=[]  NoiseDistribution=none  NoiseParameters=[]  Unit=V*A  AffineConversion=off  FilteringAndDerivatives=provide  SimscapeFilterOrder=1  InputFilterTimeConstant=0.001  UdotUserProvided=0
  Variable Resistor : fl_lib/Electrical/Electrical Elements/Variable Resistor  Rmin=0 Ohm  i_specify=off  i_priority=None  i=0 A  i_nominal_specify=off  i_nominal_unit=A  i_nominal_value=1  v_specify=off  v_priority=None  v=0 V  v_nominal_specify=off  v_nominal_unit=V  v_nominal_value=1
  Vnom : fl_lib/Physical Signals/Sources/PS Constant  constant=Vnom V
  Voltage Sensor : fl_lib/Electrical/Electrical Sensors/Voltage Sensor
  IndustrialOut : PMIOPort  Side=Right
  tag scope: Residential_power13=global
  wires:
  Repeating Sequence Interpolated3/1 -> MATLAB Function/8(data4)
  Repeating Sequence Interpolated2/1 -> MATLAB Function/7(data3)
  Repeating Sequence Interpolated1/1 -> MATLAB Function/6(data2)
  Repeating Sequence Interpolated/1 -> MATLAB Function/5(data1)
  [Button1selected] -> MATLAB Function/1(button1)
  [Button2selected] -> MATLAB Function/2(button2)
  [Button3selected] -> MATLAB Function/3(button3)
  [Button4selected] -> MATLAB Function/4(button4)
  Product/1 -> [Residential_power13]  "power"
  PS-Simulink Converter1/1 -> Product/1  "current"
  PS-Simulink Converter/1 -> Product/2  "voltage"
  MATLAB Function/1(y) -> Simulink-PS Converter1/1, Scope/1  "electrical"
  connections:
  Current Sensor/LConn1 -- Simscape Bus1/LConn1
  Current Sensor/RConn1 -- PS-Simulink Converter1/LConn1
  Voltage Sensor/RConn1 -- PS-Simulink Converter/LConn1
  Current Sensor/RConn2 -- Variable Resistor/LConn2 -- Voltage Sensor/LConn1
  IndustrialOut/RConn1 -- Simscape Bus1/RConn1
  Variable Resistor/RConn1 -- Simscape Bus1/LConn2 -- Voltage Sensor/RConn2
  Vnom/RConn1 -- PS Product/LConn2 -- PS Product/LConn1
  PS Divide/LConn2 -- Simulink-PS Converter1/RConn1
  Variable Resistor/LConn1 -- PS Divide/RConn1
  PS Divide/LConn1 -- PS Product/RConn1

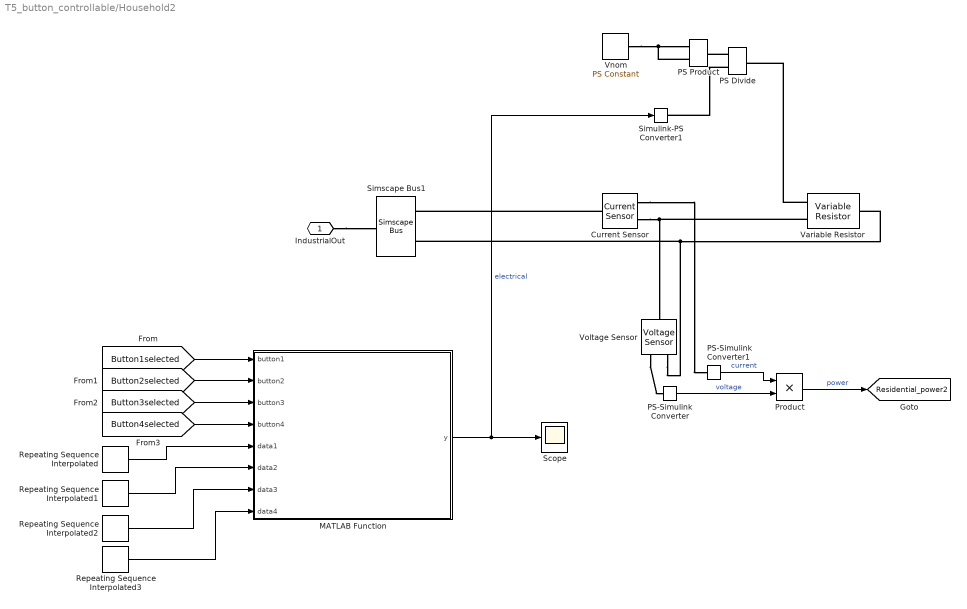
== system T5_button_controllable/Household2 ==
  Current Sensor : fl_lib/Electrical/Electrical Sensors/Current Sensor
  MATLAB Function : MATLAB Function  TreatAsAtomicUnit=on
  PS Divide : fl_lib/Physical Signals/Functions/PS Divide
  PS Product : fl_lib/Physical Signals/Functions/PS Product
  PS-Simulink Converter : nesl_utility/PS-Simulink Converter  PhysicalDomain=network_engine_domain  SubClassName=ps_output  LeftPortType=input  RightPortType=output  PseudoPeriodic=off  Frequencies=[]  VectorFormat=inherit  Unit=inherit  AffineConversion=off
  PS-Simulink Converter1 : nesl_utility/PS-Simulink Converter  PhysicalDomain=network_engine_domain  SubClassName=ps_output  LeftPortType=input  RightPortType=output  PseudoPeriodic=off  Frequencies=[]  VectorFormat=inherit  Unit=inherit  AffineConversion=off
  Product : Product
  Repeating Sequence Interpolated : simulink/Sources/Repeating Sequence Interpolated  OutValues=Household15_Springallday  TimeValues=Allday_timevector  LookUpMeth=Interpolation-Use End Values  tsamp=0.01  OutMin=[]  OutMax=[]  OutDataTypeStr=double  OutputDataTypeScalingMode=double  OutDataType=fixdt(0,8)  OutScaling=2^-10
  Repeating Sequence Interpolated1 : simulink/Sources/Repeating Sequence Interpolated  OutValues=Household15_Summerallday  TimeValues=Allday_timevector  LookUpMeth=Interpolation-Use End Values  tsamp=0.01  OutMin=[]  OutMax=[]  OutDataTypeStr=double  OutputDataTypeScalingMode=double  OutDataType=fixdt(0,8)  OutScaling=2^-10
  Repeating Sequence Interpolated2 : simulink/Sources/Repeating Sequence Interpolated  OutValues=Household15_Autumnallday  TimeValues=Allday_timevector  LookUpMeth=Interpolation-Use End Values  tsamp=0.01  OutMin=[]  OutMax=[]  OutDataTypeStr=double  OutputDataTypeScalingMode=double  OutDataType=fixdt(0,8)  OutScaling=2^-10
  Repeating Sequence Interpolated3 : simulink/Sources/Repeating Sequence Interpolated  OutValues=Household15_Winterallday  TimeValues=Allday_timevector  LookUpMeth=Interpolation-Use End Values  tsamp=0.01  OutMin=[]  OutMax=[]  OutDataTypeStr=double  OutputDataTypeScalingMode=double  OutDataType=fixdt(0,8)  OutScaling=2^-10
  Scope : Scope
  Simscape Bus1 : SimscapeBus  HierarchyStrings=High;Low
  Simulink-PS Converter1 : nesl_utility/Simulink-PS Converter  PhysicalDomain=network_engine_domain  SubClassName=ps_input  LeftPortType=input  RightPortType=output  PseudoPeriodic=off  Frequencies=[]  NoiseDistribution=none  NoiseParameters=[]  Unit=V*A  AffineConversion=off  FilteringAndDerivatives=provide  SimscapeFilterOrder=1  InputFilterTimeConstant=0.001  UdotUserProvided=0
  Variable Resistor : fl_lib/Electrical/Electrical Elements/Variable Resistor  Rmin=0 Ohm  i_specify=off  i_priority=None  i=0 A  i_nominal_specify=off  i_nominal_unit=A  i_nominal_value=1  v_specify=off  v_priority=None  v=0 V  v_nominal_specify=off  v_nominal_unit=V  v_nominal_value=1
  Vnom : fl_lib/Physical Signals/Sources/PS Constant  constant=Vnom V
  Voltage Sensor : fl_lib/Electrical/Electrical Sensors/Voltage Sensor
  IndustrialOut : PMIOPort  Side=Right
  tag scope: Residential_power2=global
  wires:
  Repeating Sequence Interpolated3/1 -> MATLAB Function/8(data4)
  Repeating Sequence Interpolated2/1 -> MATLAB Function/7(data3)
  Repeating Sequence Interpolated1/1 -> MATLAB Function/6(data2)
  Repeating Sequence Interpolated/1 -> MATLAB Function/5(data1)
  [Button1selected] -> MATLAB Function/1(button1)
  [Button2selected] -> MATLAB Function/2(button2)
  [Button3selected] -> MATLAB Function/3(button3)
  [Button4selected] -> MATLAB Function/4(button4)
  Product/1 -> [Residential_power2]  "power"
  PS-Simulink Converter1/1 -> Product/1  "current"
  PS-Simulink Converter/1 -> Product/2  "voltage"
  MATLAB Function/1(y) -> Simulink-PS Converter1/1, Scope/1  "electrical"
  connections:
  Current Sensor/LConn1 -- Simscape Bus1/LConn1
  Current Sensor/RConn1 -- PS-Simulink Converter1/LConn1
  Voltage Sensor/RConn1 -- PS-Simulink Converter/LConn1
  Current Sensor/RConn2 -- Variable Resistor/LConn2 -- Voltage Sensor/LConn1
  IndustrialOut/RConn1 -- Simscape Bus1/RConn1
  Variable Resistor/RConn1 -- Simscape Bus1/LConn2 -- Voltage Sensor/RConn2
  Vnom/RConn1 -- PS Product/LConn2 -- PS Product/LConn1
  PS Divide/LConn2 -- Simulink-PS Converter1/RConn1
  Variable Resistor/LConn1 -- PS Divide/RConn1
  PS Divide/LConn1 -- PS Product/RConn1

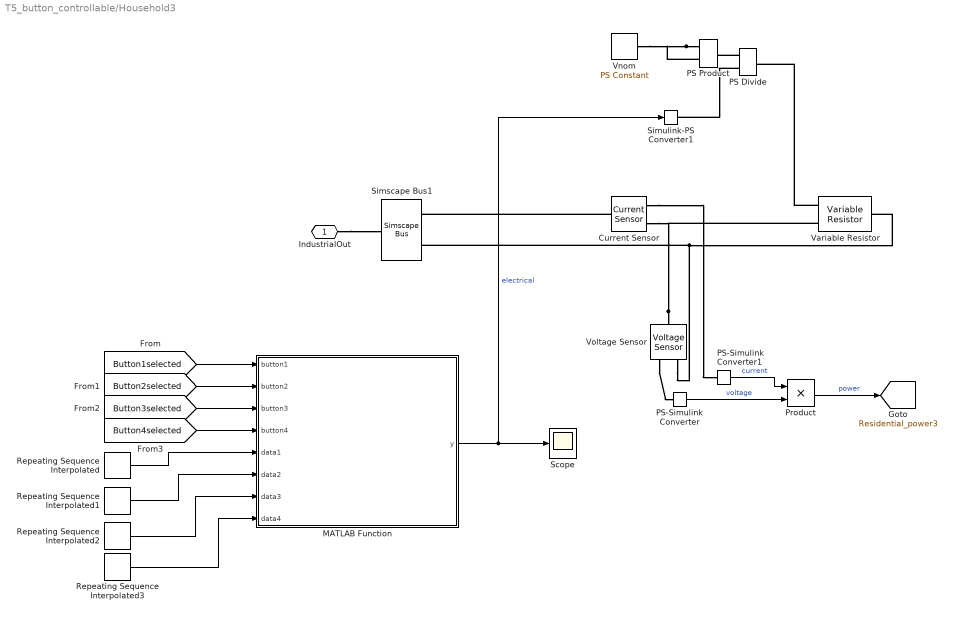
== system T5_button_controllable/Household3 ==
  Current Sensor : fl_lib/Electrical/Electrical Sensors/Current Sensor
  MATLAB Function : MATLAB Function  TreatAsAtomicUnit=on
  PS Divide : fl_lib/Physical Signals/Functions/PS Divide
  PS Product : fl_lib/Physical Signals/Functions/PS Product
  PS-Simulink Converter : nesl_utility/PS-Simulink Converter  PhysicalDomain=network_engine_domain  SubClassName=ps_output  LeftPortType=input  RightPortType=output  PseudoPeriodic=off  Frequencies=[]  VectorFormat=inherit  Unit=inherit  AffineConversion=off
  PS-Simulink Converter1 : nesl_utility/PS-Simulink Converter  PhysicalDomain=network_engine_domain  SubClassName=ps_output  LeftPortType=input  RightPortType=output  PseudoPeriodic=off  Frequencies=[]  VectorFormat=inherit  Unit=inherit  AffineConversion=off
  Product : Product
  Repeating Sequence Interpolated : simulink/Sources/Repeating Sequence Interpolated  OutValues=Household8_Springallday  TimeValues=Allday_timevector  LookUpMeth=Interpolation-Use End Values  tsamp=0.01  OutMin=[]  OutMax=[]  OutDataTypeStr=double  OutputDataTypeScalingMode=double  OutDataType=fixdt(0,8)  OutScaling=2^-10
  Repeating Sequence Interpolated1 : simulink/Sources/Repeating Sequence Interpolated  OutValues=Household8_Summerallday  TimeValues=Allday_timevector  LookUpMeth=Interpolation-Use End Values  tsamp=0.01  OutMin=[]  OutMax=[]  OutDataTypeStr=double  OutputDataTypeScalingMode=double  OutDataType=fixdt(0,8)  OutScaling=2^-10
  Repeating Sequence Interpolated2 : simulink/Sources/Repeating Sequence Interpolated  OutValues=Household8_Autumnallday  TimeValues=Allday_timevector  LookUpMeth=Interpolation-Use End Values  tsamp=0.01  OutMin=[]  OutMax=[]  OutDataTypeStr=double  OutputDataTypeScalingMode=double  OutDataType=fixdt(0,8)  OutScaling=2^-10
  Repeating Sequence Interpolated3 : simulink/Sources/Repeating Sequence Interpolated  OutValues=Household8_Winterallday  TimeValues=Allday_timevector  LookUpMeth=Interpolation-Use End Values  tsamp=0.01  OutMin=[]  OutMax=[]  OutDataTypeStr=double  OutputDataTypeScalingMode=double  OutDataType=fixdt(0,8)  OutScaling=2^-10
  Scope : Scope
  Simscape Bus1 : SimscapeBus  HierarchyStrings=High;Low
  Simulink-PS Converter1 : nesl_utility/Simulink-PS Converter  PhysicalDomain=network_engine_domain  SubClassName=ps_input  LeftPortType=input  RightPortType=output  PseudoPeriodic=off  Frequencies=[]  NoiseDistribution=none  NoiseParameters=[]  Unit=V*A  AffineConversion=off  FilteringAndDerivatives=provide  SimscapeFilterOrder=1  InputFilterTimeConstant=0.001  UdotUserProvided=0
  Variable Resistor : fl_lib/Electrical/Electrical Elements/Variable Resistor  Rmin=0 Ohm  i_specify=off  i_priority=None  i=0 A  i_nominal_specify=off  i_nominal_unit=A  i_nominal_value=1  v_specify=off  v_priority=None  v=0 V  v_nominal_specify=off  v_nominal_unit=V  v_nominal_value=1
  Vnom : fl_lib/Physical Signals/Sources/PS Constant  constant=Vnom V
  Voltage Sensor : fl_lib/Electrical/Electrical Sensors/Voltage Sensor
  IndustrialOut : PMIOPort  Side=Right
  tag scope: Residential_power3=global
  wires:
  MATLAB Function/1(y) -> Simulink-PS Converter1/1, Scope/1  "electrical"
  PS-Simulink Converter/1 -> Product/2  "voltage"
  PS-Simulink Converter1/1 -> Product/1  "current"
  Product/1 -> [Residential_power3]  "power"
  [Button4selected] -> MATLAB Function/4(button4)
  [Button3selected] -> MATLAB Function/3(button3)
  [Button2selected] -> MATLAB Function/2(button2)
  [Button1selected] -> MATLAB Function/1(button1)
  Repeating Sequence Interpolated/1 -> MATLAB Function/5(data1)
  Repeating Sequence Interpolated1/1 -> MATLAB Function/6(data2)
  Repeating Sequence Interpolated2/1 -> MATLAB Function/7(data3)
  Repeating Sequence Interpolated3/1 -> MATLAB Function/8(data4)
  connections:
  PS Divide/LConn1 -- PS Product/RConn1
  Variable Resistor/LConn1 -- PS Divide/RConn1
  PS Divide/LConn2 -- Simulink-PS Converter1/RConn1
  PS Product/LConn1 -- PS Product/LConn2 -- Vnom/RConn1
  Voltage Sensor/RConn2 -- Simscape Bus1/LConn2 -- Variable Resistor/RConn1
  IndustrialOut/RConn1 -- Simscape Bus1/RConn1
  Voltage Sensor/LConn1 -- Variable Resistor/LConn2 -- Current Sensor/RConn2
  Voltage Sensor/RConn1 -- PS-Simulink Converter/LConn1
  Current Sensor/RConn1 -- PS-Simulink Converter1/LConn1
  Current Sensor/LConn1 -- Simscape Bus1/LConn1

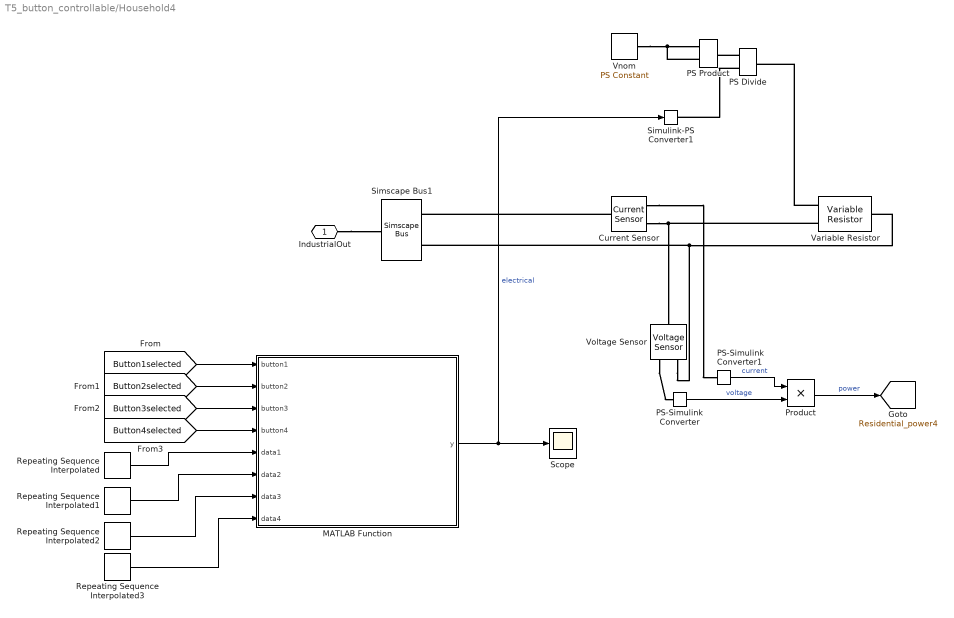
== system T5_button_controllable/Household4 ==
  Current Sensor : fl_lib/Electrical/Electrical Sensors/Current Sensor
  MATLAB Function : MATLAB Function  TreatAsAtomicUnit=on
  PS Divide : fl_lib/Physical Signals/Functions/PS Divide
  PS Product : fl_lib/Physical Signals/Functions/PS Product
  PS-Simulink Converter : nesl_utility/PS-Simulink Converter  PhysicalDomain=network_engine_domain  SubClassName=ps_output  LeftPortType=input  RightPortType=output  PseudoPeriodic=off  Frequencies=[]  VectorFormat=inherit  Unit=inherit  AffineConversion=off
  PS-Simulink Converter1 : nesl_utility/PS-Simulink Converter  PhysicalDomain=network_engine_domain  SubClassName=ps_output  LeftPortType=input  RightPortType=output  PseudoPeriodic=off  Frequencies=[]  VectorFormat=inherit  Unit=inherit  AffineConversion=off
  Product : Product
  Repeating Sequence Interpolated : simulink/Sources/Repeating Sequence Interpolated  OutValues=Household4_Springallday  TimeValues=Allday_timevector  LookUpMeth=Interpolation-Use End Values  tsamp=0.01  OutMin=[]  OutMax=[]  OutDataTypeStr=double  OutputDataTypeScalingMode=double  OutDataType=fixdt(0,8)  OutScaling=2^-10
  Repeating Sequence Interpolated1 : simulink/Sources/Repeating Sequence Interpolated  OutValues=Household4_Summerallday  TimeValues=Allday_timevector  LookUpMeth=Interpolation-Use End Values  tsamp=0.01  OutMin=[]  OutMax=[]  OutDataTypeStr=double  OutputDataTypeScalingMode=double  OutDataType=fixdt(0,8)  OutScaling=2^-10
  Repeating Sequence Interpolated2 : simulink/Sources/Repeating Sequence Interpolated  OutValues=Household4_Autumnallday  TimeValues=Allday_timevector  LookUpMeth=Interpolation-Use End Values  tsamp=0.01  OutMin=[]  OutMax=[]  OutDataTypeStr=double  OutputDataTypeScalingMode=double  OutDataType=fixdt(0,8)  OutScaling=2^-10
  Repeating Sequence Interpolated3 : simulink/Sources/Repeating Sequence Interpolated  OutValues=Household4_Winterallday  TimeValues=Allday_timevector  LookUpMeth=Interpolation-Use End Values  tsamp=0.01  OutMin=[]  OutMax=[]  OutDataTypeStr=double  OutputDataTypeScalingMode=double  OutDataType=fixdt(0,8)  OutScaling=2^-10
  Scope : Scope
  Simscape Bus1 : SimscapeBus  HierarchyStrings=High;Low
  Simulink-PS Converter1 : nesl_utility/Simulink-PS Converter  PhysicalDomain=network_engine_domain  SubClassName=ps_input  LeftPortType=input  RightPortType=output  PseudoPeriodic=off  Frequencies=[]  NoiseDistribution=none  NoiseParameters=[]  Unit=V*A  AffineConversion=off  FilteringAndDerivatives=provide  SimscapeFilterOrder=1  InputFilterTimeConstant=0.001  UdotUserProvided=0
  Variable Resistor : fl_lib/Electrical/Electrical Elements/Variable Resistor  Rmin=0 Ohm  i_specify=off  i_priority=None  i=0 A  i_nominal_specify=off  i_nominal_unit=A  i_nominal_value=1  v_specify=off  v_priority=None  v=0 V  v_nominal_specify=off  v_nominal_unit=V  v_nominal_value=1
  Vnom : fl_lib/Physical Signals/Sources/PS Constant  constant=Vnom V
  Voltage Sensor : fl_lib/Electrical/Electrical Sensors/Voltage Sensor
  IndustrialOut : PMIOPort  Side=Right
  tag scope: Residential_power4=global
  wires:
  Repeating Sequence Interpolated3/1 -> MATLAB Function/8(data4)
  Repeating Sequence Interpolated2/1 -> MATLAB Function/7(data3)
  Repeating Sequence Interpolated1/1 -> MATLAB Function/6(data2)
  Repeating Sequence Interpolated/1 -> MATLAB Function/5(data1)
  [Button1selected] -> MATLAB Function/1(button1)
  [Button2selected] -> MATLAB Function/2(button2)
  [Button3selected] -> MATLAB Function/3(button3)
  [Button4selected] -> MATLAB Function/4(button4)
  Product/1 -> [Residential_power4]  "power"
  PS-Simulink Converter1/1 -> Product/1  "current"
  PS-Simulink Converter/1 -> Product/2  "voltage"
  MATLAB Function/1(y) -> Simulink-PS Converter1/1, Scope/1  "electrical"
  connections:
  Current Sensor/LConn1 -- Simscape Bus1/LConn1
  Current Sensor/RConn1 -- PS-Simulink Converter1/LConn1
  Voltage Sensor/RConn1 -- PS-Simulink Converter/LConn1
  Current Sensor/RConn2 -- Variable Resistor/LConn2 -- Voltage Sensor/LConn1
  IndustrialOut/RConn1 -- Simscape Bus1/RConn1
  Variable Resistor/RConn1 -- Simscape Bus1/LConn2 -- Voltage Sensor/RConn2
  Vnom/RConn1 -- PS Product/LConn2 -- PS Product/LConn1
  PS Divide/LConn2 -- Simulink-PS Converter1/RConn1
  Variable Resistor/LConn1 -- PS Divide/RConn1
  PS Divide/LConn1 -- PS Product/RConn1
